simulink model "Induction Machine"  (R2020b)
settings: Solver=ode23tb  StartTime=0  StopTime=.8  MaxStep=.001  RelTol=1e-3  EnableMultiTasking=on
libraries: powerlib x9, powerlib_meascontrol x4
settings Model: Creator=Jayanti  LastModifiedBy=talha
settings DataIOCC: FinalStateName=xInitial  LimitDataPoints=on  SaveFinalState=on  SaveFormat=Array  SignalLoggingSaveFormat=ModelDataLogs  SaveOutput=off  SaveTime=off  ReturnWorkspaceOutputs=off
settings OptimizationCC: ExpressionDepthLimit=2147483647  InitFltsAndDblsToZero=on  LifeSpan=inf
settings DebuggingCC: SaveWithParameterizedLinksMsg=none  UnderspecifiedInitializationDetection=Classic  MergeDetectMultiDrivingBlocksExec=none  SignalResolutionControl=TryResolveAllWithWarning  SolverPrmCheckMsg=warning  MultiTaskDSMMsg=warning  MultiTaskCondExecSysMsg=none  FcnCallInpInsideContextMsg=warning  StateNameClashWarn=warning  SFUnexpectedBacktrackingDiag=warning  SFNoUnconditionalDefaultTransitionDiag=warning  ArithmeticOperatorsInVariantConditions=warning
settings HardwareCC: ProdBitPerPointer=32  ProdBitPerSizeT=32  ProdBitPerPtrDiffT=32  ProdLargestAtomicFloat=None  ProdIntDivRoundTo=Undefined  ProdEndianess=Unspecified  ProdWordSize=32  ProdHWDeviceType=32-bit Generic
settings ModelReferenceCC: PropagateSignalLabelsOutOfModel=off
settings SFSimCC: SimUseLocalCustomCode=off  CustomCodeUndefinedFunction=UseInterfaceOnly
settings RTWCC: RTWUseLocalCustomCode=off
settings CodeAppCC: StateflowObjectComments=on
settings GRTTargetCC: TargetFcnLib=ansi_tfl_tmw.mat  TargetLangStandard=C89/C90 (ANSI)  CombineOutputUpdateFcns=off  GRTInterface=on
settings ConfigComp: CovMetricSettings=dw  CovSaveCumulativeToWorkspaceVar=on  CovSaveSingleToWorkspaceVar=on  CovExternalEMLEnable=off  CovSFcnEnable=off
settings SimscapeCC: SimscapeNormalizeSystem=off

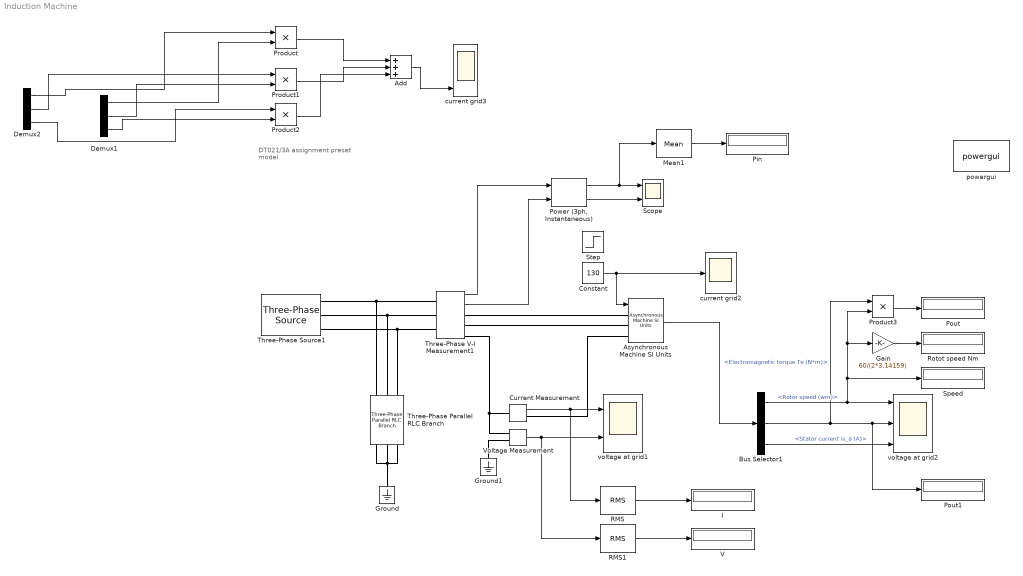
== system Induction Machine ==
  note: DT021/3A assignment
      |
      |  preset model
  " current grid2" : Scope
  " current grid3" : Scope  NumInputPorts=3
  Add : Sum  Inputs=+++
  Asynchronous Machine SI Units : powerlib/Machines/Asynchronous Machine SI Units  RotorType=Squirrel-cage  PresetModel="21:  215 HP (160KW) 400 V 50Hz 1487 RPM"  MechanicalLoad=Speed w  ShowDetailedParameters=on  ReferenceFrame=Rotor  Units=SI  MeasurementBus=off  NominalParameters=[1.6e+05 400 50]  Stator=[0.01379 0.000152]  Rotor=[0.007728 0.000152]  Cage1=[0.4155 0.002066]  Cage2=[0.4168 0.0003495]  Lm=0.00769  Mechanical=[2.9 0.05658 2]  PolePairs=2  InitialConditions=[0 0 0 0 0 0 0 0]  SimulateSaturation=off  Saturation=[14.03593122, 27.81365428, 53.79336849, 72.68890987, 97.98006896, 148.6815601, 215.7428561, 302.9841135, 428.7778367 ; 230, 322, 414, 460, 506, 552, 598, 644, 690]  LoadFlowParameters=1492000  TsPowergui=0  TsBlock=-1  IterativeModel=Trapezoidal non iterative  IterativeDiscreteModel=Trapezoidal non iterative  Pmec=1.492e+006
  Bus Selector1 : BusSelector  OutputSignals=Mechanical.Rotor speed (wm),Mechanical.Electromagnetic torque Te (N*m),Stator measurements.Stator current is_a (A)
  Constant : Constant  Value=130
  Current Measurement : powerlib/Measurements/Current Measurement  PhasorSimulation=off  OutputType=Complex  PSBequivalent=0
  Demux1 : Demux  Outputs=3
  Demux2 : Demux  Outputs=3
  Gain : Gain  Gain=60/(2*3.14159)
  Ground : powerlib/Elements/Ground  LConnTagsString=a
  Ground1 : powerlib/Elements/Ground  LConnTagsString=a
  I : Display
  Mean1 : powerlib_meascontrol/Measurements/Mean  Freq=50  Vinit=0  Ts=0
  Pin : Display
  Pout : Display
  Pout1 : Display
  "Power (3ph, Instantaneous)" : powerlib_meascontrol/Measurements/Power (3ph, Instantaneous)
  Product{,1..3} (4 alike) : Product
  RMS : powerlib_meascontrol/Measurements/RMS  TrueRMS=on  Freq=50  RMSInit=120  Ts=0
  RMS1 : powerlib_meascontrol/Measurements/RMS  TrueRMS=on  Freq=50  RMSInit=120  Ts=0
  Rotot speed Nm : Display
  Scope : Scope  NumInputPorts=2
  Speed : Display
  Step : Step  Time=.3  Before=7  After=25  SampleTime=0
  Three-Phase Parallel RLC Branch : powerlib/Elements/Three-Phase Parallel RLC Branch  LConnTagsString=A|B|C  RConnTagsString=A|B|C  BranchType=R  Resistance=100e6  Inductance=1e-3  Capacitance=1e-6  Measurements=None
      settings: SourceProductBaseCode=PS
  Three-Phase V-I Measurement1 : powerlib/Measurements/Three-Phase V-I Measurement  VoltageMeasurement=phase-to-ground  SetLabelV=off  LabelV=Vabc  Vpu=off  VpuLL=off  CurrentMeasurement=yes  SetLabelI=off  LabelI=Iabc  Ipu=off  Pbase=100e6  Vbase=500e3  OutputType=Complex  PhasorSimulation=off  PSBequivalent=0
  Three-Phase Source1 : powerlib/Electrical Sources/Three-Phase Source  InternalConnection=Yg  VoltagePhases=off  Voltage=400  PhaseAngle=0  Voltage_phases=[400 400 400]/sqrt(3)  PhaseAngles_phases=[0 -120 +120]  Frequency=50  NonIdealSource=off  SpecifyImpedance=on  Resistance=0.8929  Inductance=16.58e-3  ShortCircuitLevel=10e6  BaseVoltage=400  XRratio=20  BusType=swing  Pref=0  Qref=0  Prefabc=[10e3, 10e3, 10e3]  Qrefabc=[0, 0, 0]  Qmin=-inf  Qmax=inf
  V : Display
  Voltage Measurement : powerlib/Measurements/Voltage Measurement  PhasorSimulation=off  OutputType=Complex  PSBequivalent=0
  powergui : powerlib/powergui  Priority=2  SimulationMode=Continuous  SampleTime=0  frequency=50  Iterations=50  frequencyindice=50  Pbase=100e6  ErrMax=1e-4  UnitsV=kV  UnitsW=MW  buscounter=0  FunctionMessages=off  echomessages=off  EnableUseOfTLC=off  CurrentSourceSwitches=off  DisableSnubberDevices=off  DisableRonSwitches=off  DisableVfSwitches=off  DisplayEquations=off  AutomaticDiscreteSolvers=off  SolverType=Tustin  Interpol=off  ExternalGateDelay=off  methode=off  Ts=0  x0status=blocks  SPID=off  SwTol=0  HookPort=off  NonlinearTolerance=1e-4  nMaxIteration=100  ContinueOnMaxIteration=off  RestoreLinks=warning  ResistiveCurrentMeasurement=off  Frange=[0:2:500]  Ylog=off  Xlog=off  ShowGrid=off  save=off  variable=ZData  structure=0  ZoomFFT=on  StartTime=0.0  cycles=1  DisplayStyle=1  fundamental=60  FreqAxis=off  MaxFrequency=1000  frequencyindicesteady=1  RmsSteady=1  display=off
  voltage at grid1 : Scope  NumInputPorts=2
  voltage at grid2 : Scope  NumInputPorts=3
  wires:
  Asynchronous Machine SI Units/1 -> Bus Selector1/1
  Current Measurement/1 -> RMS/1, voltage at grid1/1
  Voltage Measurement/1 -> RMS1/1, voltage at grid1/2
  Bus Selector1/3 -> voltage at grid2/3  "<Stator current is_a (A)>"
  Bus Selector1/1 -> Product3/2, Gain/1, Speed/1, voltage at grid2/1  "<Rotor speed (wm)>"
  Bus Selector1/2 -> Product3/1, Pout1/1, voltage at grid2/2  "<Electromagnetic torque Te (N*m)>"
  Demux2/1 -> Product/1
  Demux1/1 -> Product/2
  Demux2/2 -> Product1/1
  Demux1/2 -> Product1/2
  Demux2/3 -> Product2/1
  Demux1/3 -> Product2/2
  Product/1 -> Add/1
  Product1/1 -> Add/2
  Product2/1 -> Add/3
  Add/1 -> " current grid3"/3
  RMS/1 -> I/1
  RMS1/1 -> V/1
  Product3/1 -> Pout/1
  Mean1/1 -> Pin/1
  Three-Phase V-I Measurement1/2 -> "Power (3ph, Instantaneous)"/2
  Three-Phase V-I Measurement1/1 -> "Power (3ph, Instantaneous)"/1
  "Power (3ph, Instantaneous)"/1 -> Mean1/1, Scope/1
  "Power (3ph, Instantaneous)"/2 -> Scope/2
  Constant/1 -> " current grid2"/1, Asynchronous Machine SI Units/1
  Gain/1 -> Rotot speed Nm/1
  connections:
  Three-Phase Source1/RConn2 -- Three-Phase V-I Measurement1/LConn2 -- Three-Phase Parallel RLC Branch/LConn2
  Three-Phase Source1/RConn1 -- Three-Phase V-I Measurement1/LConn1 -- Three-Phase Parallel RLC Branch/LConn1
  Three-Phase Source1/RConn3 -- Three-Phase V-I Measurement1/LConn3 -- Three-Phase Parallel RLC Branch/LConn3
  Asynchronous Machine SI Units/LConn2 -- Three-Phase V-I Measurement1/RConn2
  Asynchronous Machine SI Units/LConn1 -- Three-Phase V-I Measurement1/RConn1
  Ground/LConn1 -- Three-Phase Parallel RLC Branch/RConn3 -- Three-Phase Parallel RLC Branch/RConn1 -- Three-Phase Parallel RLC Branch/RConn2
  Current Measurement/LConn1 -- Voltage Measurement/LConn1 -- Three-Phase V-I Measurement1/RConn3
  Asynchronous Machine SI Units/LConn3 -- Current Measurement/RConn1
  Voltage Measurement/LConn2 -- Ground1/LConn1
